simulink model "TST_AdvancedStateflowLoops3"  (Simulink 10.0)
settings: Solver=FixedStepDiscrete  StartTime=0.0  StopTime=10.0  FixedStep=0.02  RelTol=1e-3  EnableMultiTasking=on
settings Model: Creator=kharthforeign  LastModifiedBy=unknown
settings DataIOCC: LimitDataPoints=on  SignalLoggingSaveFormat=ModelDataLogs  SaveOutput=off  SignalLogging=off  SaveTime=off
settings OptimizationCC: BlockReduction=off  ConditionallyExecuteInputs=off  OptimizeBlockIOStorage=off  BufferReuse=off  GlobalBufferReuse=off  ExpressionFolding=off  ExpressionDepthLimit=2147483647  LocalBlockOutputs=off  InitFltsAndDblsToZero=on  OptimizeDataStoreBuffers=off  BusAssignmentInplaceUpdate=off
settings DebuggingCC: SolverPrmCheckMsg=warning  FcnCallInpInsideContextMsg=warning  StateNameClashWarn=warning
settings SFSimCC: SimParseCustomCode=off
settings GRTTargetCC: GeneratePreprocessorConditionals=Disable all
settings ConfigComp: CovExternalEMLEnable=off

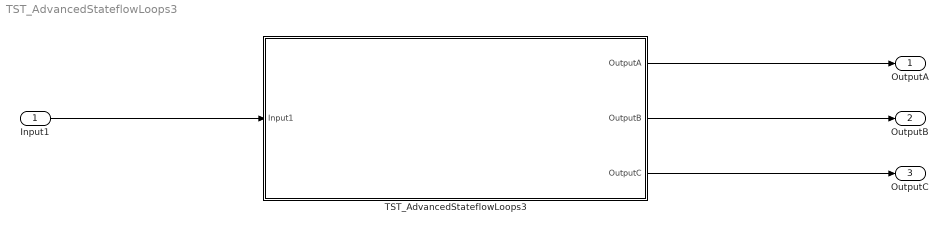
== system TST_AdvancedStateflowLoops3 ==
  Input1 : Inport  OutDataTypeStr=uint32  BusOutputAsStruct=on
  TST_AdvancedStateflowLoops3 : Subsystem  TreatAsAtomicUnit=on
  OutputA : Outport  OutDataTypeStr=double  PortDimensions=1
  OutputB : Outport  Port=2  OutDataTypeStr=double  PortDimensions=1
  OutputC : Outport  Port=3  OutDataTypeStr=double  PortDimensions=1
  wires:
  Input1/1 -> TST_AdvancedStateflowLoops3/1(Input1)
  TST_AdvancedStateflowLoops3/1(OutputA) -> OutputA/1
  TST_AdvancedStateflowLoops3/2(OutputB) -> OutputB/1
  TST_AdvancedStateflowLoops3/3(OutputC) -> OutputC/1

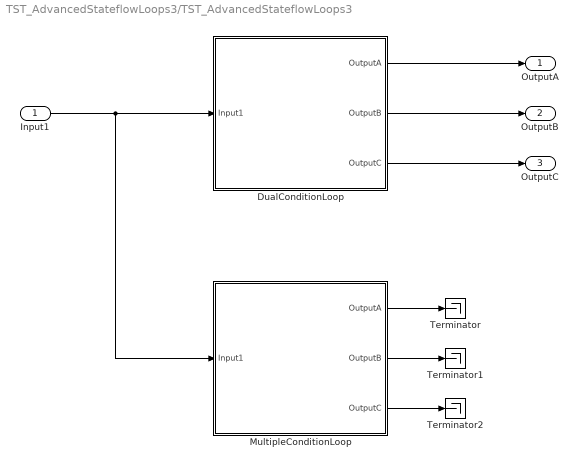
== system TST_AdvancedStateflowLoops3/TST_AdvancedStateflowLoops3 ==
  Input1 : Inport  OutDataTypeStr=uint32  BusOutputAsStruct=on
  DualConditionLoop : Stateflow chart  TreatAsAtomicUnit=on
  MultipleConditionLoop : Stateflow chart  TreatAsAtomicUnit=on
  Terminator : Terminator
  Terminator1 : Terminator
  Terminator2 : Terminator
  OutputA : Outport  OutDataTypeStr=double  PortDimensions=1
  OutputB : Outport  Port=2  OutDataTypeStr=double  PortDimensions=1
  OutputC : Outport  Port=3  OutDataTypeStr=double  PortDimensions=1
  wires:
  DualConditionLoop/1(OutputA) -> OutputA/1
  DualConditionLoop/2(OutputB) -> OutputB/1
  DualConditionLoop/3(OutputC) -> OutputC/1
  Input1/1 -> DualConditionLoop/1(Input1), MultipleConditionLoop/1(Input1)
  MultipleConditionLoop/1(OutputA) -> Terminator/1
  MultipleConditionLoop/2(OutputB) -> Terminator1/1
  MultipleConditionLoop/3(OutputC) -> Terminator2/1

== stateflow chart TST_AdvancedStateflowLoops3/MultipleConditionLoop ==
  note: This flowgraph demonstrates three single-transition loops.
      | Semantically they all are part of the same repeat statement.
  (default) -> (junction 14)
  (junction 14) -> (junction 13) [order 4] : {OutputC = 99.0}
  (junction 14) -> (junction 14) [order 3] : [C]{OutputC += 3.0}
  (junction 14) -> (junction 14) [order 1] : [A]{OutputA += 1.0}
  (junction 14) -> (junction 14) [order 2] : [B]{OutputB += 2.0}
  data: Input1 input uint32; OutputA output double =1; OutputB output double =2; OutputC output double =3; Local local uint32 =0; A local boolean; B local boolean; C local boolean; D local boolean

== stateflow chart TST_AdvancedStateflowLoops3/DualConditionLoop ==
  state StateX
  note: This flowgraph demonstrates two indiviual loops that are semantically joined.
      | Because they have the same loop source/destination junction, they are
      | part of the same repeat statement.
  (default) -> (junction 34)
  (junction 34) -> StateX [order 3] : {OutputC = 7.0}
  (junction 33) -> (junction 34) : {OutputA += 2.0}
  (junction 34) -> (junction 33) [order 1] : [A]
  (junction 34) -> (junction 35) [order 2] : [B]
  (junction 35) -> (junction 34) : {OutputB += 2.0}
  data: Input1 input uint32; OutputA output double =1; OutputB output double =2; OutputC output double =3; Local local uint32 =0; A local boolean; B local boolean; C local boolean; D local boolean
